simulink model "CLFeedback"  (R2022a)
settings: Solver=VariableStepAuto  StartTime=0.0  StopTime=10.0  RelTol=1e-3
values from neighbouring files (symbols this model uses):
  F = inv(CMin*inv(-AMin+BMin*K)*BMin)    [Main.m]
  K = place(AMin,BMin,poles)    [Main.m]
undefined symbols (not defined in the file or in its folder): AMin, BMin, CMin, DMin, tau_threshold
settings Model: Creator=angelhoffman  LastModifiedBy=angelhoffman

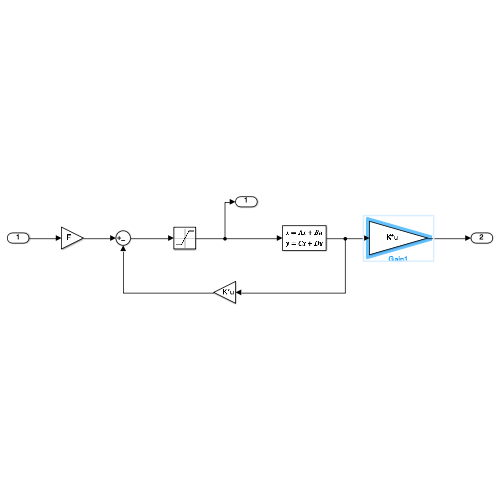
[thumbnail: Simulink's stored preview of the top-level diagram]
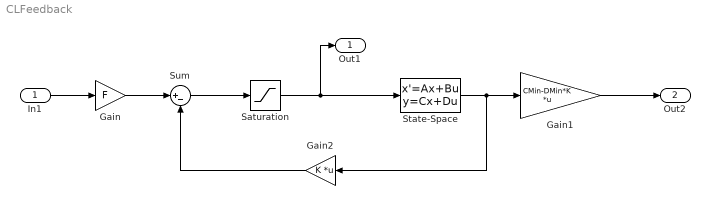
== system CLFeedback ==
  In1 : Inport
  Gain : Gain  Gain=F
  Gain1 : Gain  Gain=CMin-DMin*K  Multiplication=Matrix(K*u)
  Gain2 : Gain  Gain=K  Multiplication=Matrix(K*u)
  Saturation : Saturate  UpperLimit=tau_threshold  LowerLimit=-tau_threshold
  State-Space : StateSpace  A=AMin  B=BMin  C=eye(4)  D=zeros(4,1)  InitialCondition=zeros(4,1)
  Sum : Sum  Inputs=|+-
  Out1 : Outport
  Out2 : Outport  Port=2
  wires:
  Gain/1 -> Sum/1
  State-Space/1 -> Gain2/1, Gain1/1
  Gain1/1 -> Out2/1
  Gain2/1 -> Sum/2
  Sum/1 -> Saturation/1
  Saturation/1 -> Out1/1, State-Space/1
  In1/1 -> Gain/1
